simulink model "velocity2force"  (R2020b)
settings: Solver=VariableStepAuto  StartTime=0.0  StopTime=10.0  RelTol=1e-3
values from neighbouring files (symbols this model uses):
  b = 1.1064*10^(-5)    (= 1.1064e-05)    [variables.m]
  d = 4.406*10^-7    (= 4.406e-07)    [variables.m]
settings Model: Creator=fiori  LastModifiedBy=fiori

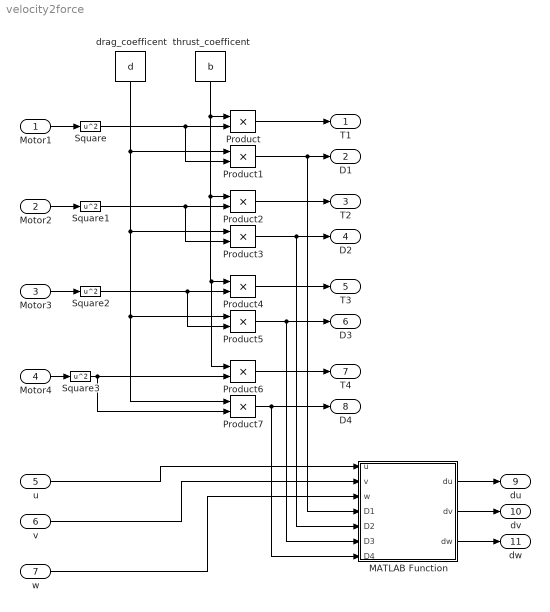
== system velocity2force ==
  Motor1 : Inport
  Motor2 : Inport  Port=2
  Motor3 : Inport  Port=3
  Motor4 : Inport  Port=4
  u : Inport  Port=5
  v : Inport  Port=6
  w : Inport  Port=7
  MATLAB Function : MATLAB Function  TreatAsAtomicUnit=on
  Product{,1..7} (8 alike) : Product
  Square{,1..3} (4 alike) : Math  Operator=square  SaturateOnIntegerOverflow=on
  drag_coefficent : Constant  Value=d
  thrust_coefficent : Constant  Value=b
  T1 : Outport
  D1 : Outport  Port=2
  T2 : Outport  Port=3
  D2 : Outport  Port=4
  T3 : Outport  Port=5
  D3 : Outport  Port=6
  T4 : Outport  Port=7
  D4 : Outport  Port=8
  du : Outport  Port=9
  dv : Outport  Port=10
  dw : Outport  Port=11
  wires:
  thrust_coefficent/1 -> Product/1, Product6/1, Product4/1, Product2/1
  Product/1 -> T1/1
  Product1/1 -> D1/1, MATLAB Function/4(D1)
  drag_coefficent/1 -> Product7/1, Product5/1, Product3/1, Product1/1
  Motor1/1 -> Square/1
  Product2/1 -> T2/1
  Product3/1 -> MATLAB Function/5(D2), D2/1
  Motor2/1 -> Square1/1
  Product4/1 -> T3/1
  Product5/1 -> MATLAB Function/6(D3), D3/1
  Product6/1 -> T4/1
  Product7/1 -> MATLAB Function/7(D4), D4/1
  Motor3/1 -> Square2/1
  Motor4/1 -> Square3/1
  Square/1 -> Product/2, Product1/2
  Square1/1 -> Product2/2, Product3/2
  Square2/1 -> Product5/2, Product4/2
  Square3/1 -> Product6/2, Product7/2
  u/1 -> MATLAB Function/1(u)
  v/1 -> MATLAB Function/2(v)
  w/1 -> MATLAB Function/3(w)
  MATLAB Function/1(du) -> du/1
  MATLAB Function/2(dv) -> dv/1
  MATLAB Function/3(dw) -> dw/1

== matlab function velocity2force/MATLAB Function ==
  data: u input; du output; v input; w input; D1 input; D2 input; D3 input; D4 input; dv output; dw output
function [du,dv,dw] = fcn(u,v,w,D1,D2,D3,D4)
D=D1+D2+D3+D4;
angolo_velocita=atan2(v,u);
angolo_su=atan2((sqrt(u^2 + v^2)),(w));
du=D*sin(angolo_su)*cos(angolo_velocita);
dv=D*sin(angolo_su)*sin(angolo_velocita);
dw=D*cos(angolo_su);
end
